simulink model "SIMQGC"  (R2017a)
settings: Solver=VariableStepAuto  StartTime=0.0  StopTime=1000  RelTol=1e-3
model workspace: external: MAT-File (data not in the file)
values from neighbouring files (symbols this model uses):
  aDe =     [MY3.mat]
  aDyn =     [MY3.mat]
  aLat =     [MY3.mat]
  aLon =     [MY3.mat]
  H = HGround + geo.Zgear + GearData.R - MCdata.mass*9.8/4/GearData.Sp    [my3_acdata.m]
  HGround = 500    [my3_acdata.m]
  phi_max = 20    [my3_acdata.m]
  phi_min = -20    [my3_acdata.m]
  psi_max = 30    [my3_acdata.m]
  psi_min = -30    [my3_acdata.m]
  theta_max = 20    [my3_acdata.m]
  theta_min = -20    [my3_acdata.m]
  Xmax = 0.01    [my3_acdata.m]
  Xmin = 0    [my3_acdata.m]
  Ymax = 0.01    [my3_acdata.m]
  Ymin = 0    [my3_acdata.m]
  Zmax = 0.01    [my3_acdata.m]
  Zmin = 0    [my3_acdata.m]
undefined symbols (not defined in the file or in its folder): Earth, geo, ini, magnitude, Motor, Newton, Prop, Raphson, Standard_Devices, UDP_Protocol, WGS84
undefined symbols (not defined in the file): GearData, LProp, RProp
libraries: simulink_extras x12, dspnetwork x8, aerolibobsolete x6, sharedutil x6, simulink x4, aerolibfltsims x3, aerolibasang x2, aerolibatmos2 x1, aerolibbdyn x1, aerolibtransform2 x1, aerolibanimutils x1, sldrtlib x1
(part 1 of 3)
settings Model: Creator=d8230  LastModifiedBy=d8230
settings SFSimCC: SimCustomInitializer=my_3acdata.m
settings RTWCC: Toolchain=Microsoft Visual C++ 2015 v14.0 | nmake (64-bit Windows)
settings CodeAppCC: ForceParamTrailComments=on  MATLABSourceComments=on

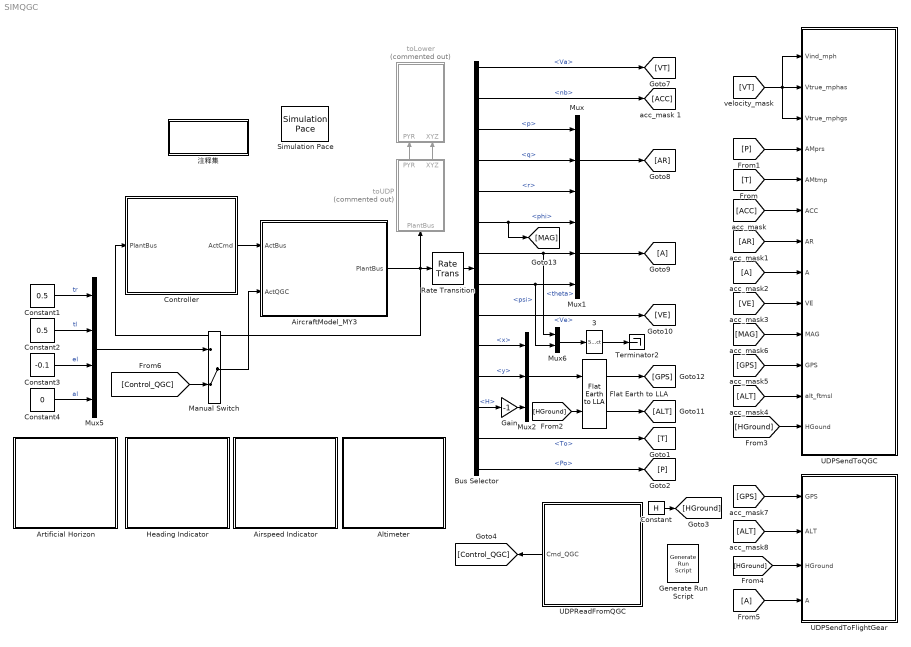
== system SIMQGC ==
  3 : Selector  InputPortWidth=2  IndexOptions=Index vector (dialog)  Indices=[2,1]  OutputSizes=1
  AircraftModel_MY3 : Subsystem
  Airspeed Indicator : Subsystem  DialogController=aeroblksHMICreateDDGDialog  IsWebBlock=on  mask(MWDashboardBlock){webBlockId=530eda5d-0ac3-4735-9d39-42895928f7ce, webBlockType=airspeedindicator, ShowInLibBrowser=on, ShowInitialText=on, HMISrcModelName=SIMQGC}
      mask prompts: webBlockId "WebBlock Id"; webBlockType "WebBlock Type"; HMISrcModelName "Source Model"
      mask help: aeroblksHMI:aeroblkhmi:AirspeedIndicatorDialogDesc
      mask Help: eval('asbhmihelp(''airspeedindicator'')');
      mask Display:
      | if strcmp(get_param(bdroot(gcb),'BlockDiagramType'), 'library')
      |  image([(matlabroot) '/toolbox/aeroblks/aeroblks/hmi/icons/AirspeedIndicatorIcon.svg'])
      | end
  Altimeter : Subsystem  DialogController=aeroblksHMICreateDDGDialog  IsWebBlock=on  mask(MWDashboardBlock){webBlockId=e81fc4a0-2f3e-46f7-8fff-bae700747e07, webBlockType=altimeter, ShowInLibBrowser=on, ShowInitialText=on, HMISrcModelName=SIMQGC}
      mask prompts: webBlockId "WebBlock Id"; webBlockType "WebBlock Type"; HMISrcModelName "Source Model"
      mask help: aeroblksHMI:aeroblkhmi:AltimeterDialogDesc
      mask Help: eval('asbhmihelp(''altimeter'')');
      mask Display:
      | if strcmp(get_param(bdroot(gcb),'BlockDiagramType'), 'library')
      |  image([(matlabroot) '/toolbox/aeroblks/aeroblks/hmi/icons/AltimeterIcon.svg'])
      | end
  Artificial Horizon : Subsystem  DialogController=aeroblksHMICreateDDGDialog  IsWebBlock=on  mask(MWDashboardBlock){webBlockId=e4013b59-c6b3-40ec-8031-c9c080829948, webBlockType=artificialhorizon, ShowInLibBrowser=on, ShowInitialText=on, HMISrcModelName=SIMQGC}
      mask prompts: webBlockId "WebBlock Id"; webBlockType "WebBlock Type"; HMISrcModelName "Source Model"
      mask help: aeroblksHMI:aeroblkhmi:ArtificialHorizonDialogDesc
      mask Help: eval('asbhmihelp(''artificialhorizon'')');
      mask Display:
      | if strcmp(get_param(bdroot(gcb),'BlockDiagramType'), 'library')
      |  image([(matlabroot) '/toolbox/aeroblks/aeroblks/hmi/icons/ArtificialHorizonIcon.svg'])
      | end
  Bus Selector : BusSelector  OutputSignals=Va,nb,p,q,r,phi,theta,psi,Ve,x,y,H,To,Po
  Constant : Constant  Value=H
  Constant1 : Constant  Value=0.5
  Constant2 : Constant  Value=0.5
  Constant3 : Constant  Value=-0.1
  Constant4 : Constant  Value=0
  Controller : Subsystem
  Flat Earth to LLA : aerolibtransform2/Flat Earth to LLA  units=Metric (MKS)  ptype=Earth (WGS84)  F=1/298.257223563  R=6378137  LL0=[34.3,108.80]  psi=0
  Gain : Gain  Gain=-1
  Generate Run Script : aerolibfltsims/Generate Run Script  OutputFileName=runfg.bat  FlightGearBaseDirectory=D:\FlightGear 3.4.0  GeometryModelName=c172p  DestinationPort=6666  OriginAddress=127.0.0.1  OriginPort=5505  LocalAddress=127.0.0.1  AirportId=KSFO  RunwayId=10L  InitialAltitude=ini.Xe(3)/0.3048  InitialHeading=0  OffsetDistance=0  OffsetAzimuth=0  GenerateFile=off  Architecture=Win64  dataFlow=Send
  Heading Indicator : Subsystem  DialogController=aeroblksHMICreateDDGDialog  IsWebBlock=on  mask(MWDashboardBlock){webBlockId=3416712c-36e7-4a0f-be9c-29638a8fd49d, webBlockType=headingindicator, ShowInLibBrowser=on, ShowInitialText=on, HMISrcModelName=SIMQGC}
      mask prompts: webBlockId "WebBlock Id"; webBlockType "WebBlock Type"; HMISrcModelName "Source Model"
      mask help: aeroblksHMI:aeroblkhmi:HeadingIndicatorDialogDesc
      mask Help: eval('asbhmihelp(''headingindicator'')');
      mask Display:
      | if strcmp(get_param(bdroot(gcb),'BlockDiagramType'), 'library')
      |  image([(matlabroot) '/toolbox/aeroblks/aeroblks/hmi/icons/HeadingIndicatorIcon.svg'])
      | end
  Manual Switch : ManualSwitch  CurrentSetting=0
  Mux : Mux  Inputs=3
  Mux1 : Mux  Inputs=3
  Mux2 : Mux  Inputs=3
  Mux5 : Mux
  Mux6 : Mux  Inputs=2
  Rate Transition : RateTransition  OutPortSampleTime=0.05
  Simulation Pace : aerolibanimutils/Simulation Pace  SimulationPace=1  SleepMode=MATLAB Thread  OutputPaceError=off  SampleTime=1/30
  Terminator2 : Terminator
  UDPReadFromQGC : Subsystem
  UDPSendToFlightGear : Subsystem
  UDPSendToQGC : Subsystem
  toLower : Subsystem  Commented=on
  toUDP : Subsystem  Commented=on
  注释集 : Subsystem
  wires:
  [P] -> UDPSendToQGC/4(AMprs)
  [T] -> UDPSendToQGC/5(AMtmp)
  [ACC] -> UDPSendToQGC/6(ACC)
  [AR] -> UDPSendToQGC/7(AR)
  [A] -> UDPSendToQGC/8(A)
  [VE] -> UDPSendToQGC/9(VE)
  [MAG] -> UDPSendToQGC/10(MAG)
  [GPS] -> UDPSendToQGC/11(GPS)
  [ALT] -> UDPSendToQGC/12(alt_ftmsl)
  [VT] -> UDPSendToQGC/1(Vind_mph), UDPSendToQGC/2(Vtrue_mphas), UDPSendToQGC/3(Vtrue_mphgs)
  Mux/1 -> [AR]
  Bus Selector/12 -> Gain/1  "<H>"
  Mux1/1 -> [A]
  Flat Earth to LLA/1 -> [GPS]
  Bus Selector/1 -> [VT]  "<Va>"
  Bus Selector/2 -> [ACC]  "<nb>"
  Bus Selector/3 -> Mux/1  "<p>"
  Bus Selector/4 -> Mux/2  "<q>"
  Bus Selector/5 -> Mux/3  "<r>"
  Bus Selector/6 -> Mux1/1, [MAG]  "<phi>"
  Bus Selector/7 -> Mux1/2, Mux6/1  "<theta>"
  Bus Selector/8 -> Mux1/3, Mux6/2  "<psi>"
  Bus Selector/9 -> [VE]  "<Ve>"
  Bus Selector/10 -> Mux2/1  "<x>"
  Bus Selector/11 -> Mux2/2  "<y>"
  Controller/1(ActCmd) -> AircraftModel_MY3/1(ActBus)
  Mux2/1 -> Flat Earth to LLA/1
  Flat Earth to LLA/2 -> [ALT]
  Gain/1 -> Mux2/3
  [HGround] -> Flat Earth to LLA/2
  toUDP/2(XYZ) -> toLower/2(XYZ)
  toUDP/1(PYR) -> toLower/1(PYR)
  AircraftModel_MY3/1(PlantBus) -> toUDP/1(PlantBus), Controller/1(PlantBus), Rate Transition/1
  Rate Transition/1 -> Bus Selector/1
  Bus Selector/13 -> [T]  "<To>"
  Bus Selector/14 -> [P]  "<Po>"
  Constant1/1 -> Mux5/1  "tr"
  Constant2/1 -> Mux5/2  "tl"
  Constant3/1 -> Mux5/3  "el"
  Constant/1 -> [HGround]
  [HGround] -> UDPSendToQGC/13("HGound ")
  [GPS] -> UDPSendToFlightGear/1(GPS)
  [ALT] -> UDPSendToFlightGear/2(ALT)
  [HGround] -> UDPSendToFlightGear/3(HGround)
  [A] -> UDPSendToFlightGear/4(A)
  3/1 -> Terminator2/1
  Mux6/1 -> 3/1
  Constant4/1 -> Mux5/4  "al"
  Manual Switch/1 -> AircraftModel_MY3/2(ActQGC)
  Mux5/1 -> Manual Switch/1
  [Control_QGC] -> Manual Switch/2
  UDPReadFromQGC/1(Cmd_QGC) -> [Control_QGC]

== system SIMQGC/AircraftModel_MY3 ==
  ActBus : Inport
  ActQGC : Inport  Port=2
  Actuator : Subsystem
  Actuator1 : Subsystem
  Bus Creator : BusCreator  Inputs=23
  Bus Selector : BusSelector  OutputSignals=dt,de,dd,da
  Constant{,1..3} (4 alike) : Constant  Value=0
  Demux : Demux
  Demux1 : Demux
  Environment : Subsystem  TreatAsAtomicUnit=on
  Fixwing_Airframe : Subsystem  TreatAsAtomicUnit=on
      mask Display:
      | port_label('output',1,'PlantData');
      | port_label('input',1,'EnvmData');
      | port_label('input',2,'ActData');
  Manual Switch : ManualSwitch  CurrentSetting=0
  Scope1 : Scope  NumInputPorts=4
  Scopes : Subsystem
  Terminator{,1..3} (4 alike) : Terminator
  outputs : Subsystem
  PlantBus : Outport
  wires:
  ActBus/1 -> Bus Selector/1
  Bus Selector/2 -> Actuator/2(de_cmd)  "<de>"
  Fixwing_Airframe/1(PlantData) -> outputs/1(Model o/p bus), Scopes/1(plant bus)
  outputs/1(p) -> Terminator3/1  "p"
  Bus Selector/3 -> Actuator/3(dd_cmd)  "<dd>"
  Environment/1(Envm) -> Fixwing_Airframe/1(EnvmData)
  Actuator/1(Airc) -> Manual Switch/1
  Bus Selector/1 -> Actuator/1(dt_cmd)  "<dt>"
  Bus Creator/1 -> PlantBus/1
  outputs/2(q) -> Bus Creator/2  "q"
  outputs/3(r) -> Terminator1/1  "r"
  outputs/4(phi) -> Terminator2/1  "phi"
  outputs/5(theta) -> Bus Creator/5  "theta"
  outputs/6(psi) -> Terminator/1  "psi"
  outputs/7(alpha) -> Bus Creator/7  "alpha"
  outputs/8(beta) -> Bus Creator/8  "beta"
  outputs/9(Va) -> Bus Creator/9  "Va"
  outputs/10(x) -> Bus Creator/10  "x"
  outputs/11(y) -> Bus Creator/11  "y"
  outputs/12(H) -> Bus Creator/12, Environment/1(H)  "H"
  outputs/13(mach) -> Bus Creator/13  "mach"
  outputs/14(gamma) -> Bus Creator/14  "gamma"
  outputs/15(chi) -> Bus Creator/15  "chi"
  outputs/16(Vy) -> Bus Creator/16  "Vy"
  outputs/17(nyb) -> Bus Creator/17  "nyb"
  outputs/18(nzb) -> Bus Creator/18  "nzb"
  outputs/19(Acc) -> Bus Creator/19  "Acc"
  outputs/20(Ve) -> Bus Creator/20  "Ve"
  ActQGC/1 -> Demux/1
  outputs/21(To) -> Bus Creator/21
  outputs/22(Po) -> Bus Creator/22
  Demux/1 -> Actuator1/1(tr_cmd)
  Demux/2 -> Actuator1/2(tl_cmd)
  Actuator1/1(Airc) -> Manual Switch/2
  Manual Switch/1 -> Demux1/1, Fixwing_Airframe/2(ActData)
  Bus Selector/4 -> Actuator/4(da_cmd)  "<da>"
  Demux/4 -> Actuator1/4(al_cmd)
  Constant/1 -> Bus Creator/6  "psi"
  Constant1/1 -> Bus Creator/3  "r"
  Constant2/1 -> Bus Creator/1  "p"
  Constant3/1 -> Bus Creator/4  "phi"
  Demux1/1 -> Scope1/1
  Demux1/2 -> Scope1/2
  Demux1/3 -> Scope1/3
  Demux1/4 -> Scope1/4
  Demux/3 -> Actuator1/3(el_cmd)
  outputs/23(nb) -> Bus Creator/23

== system SIMQGC/Airspeed Indicator ==

== system SIMQGC/Altimeter ==

== system SIMQGC/Artificial Horizon ==

== system SIMQGC/Controller ==
  PlantBus : Inport
  Add : Sum  Inputs=|+-
  Bus Creator : BusCreator  Inputs=4
  Bus Selector : BusSelector  OutputSignals=Va,gamma,H,theta,q,y,phi,p,nyb,r,psi
  Constant : Constant  Value=0
  Constant1 : Constant  Value=0
  Constant2 : Constant  Value=-600
  Gain{1,3..5} (4 alike) : Gain  Gain=1/57.3
  Gain2 : Gain  Gain=9.8
  Gain6 : Gain
  MATLAB Function : MATLAB Function  TreatAsAtomicUnit=on
  Memory1 : Memory
  RAH : Subsystem  mask{Kphi=1, Kp=3, Kr=1.4, Kff_phi=0.2, Kay=0, Kpi=0.5}
  Subsystem : Subsystem
  Terminator : Terminator
  Terminator1 : Terminator
  height_hold : Subsystem
  theta_hold : Subsystem
  v_hold1 : Subsystem
  ActCmd : Outport
  wires:
  Bus Creator/1 -> ActCmd/1  "ActCmd"
  PlantBus/1 -> Bus Selector/1
  v_hold1/1(tg) -> [dt]  "dt"
  theta_hold/1(de) -> [de]  "de"
  Bus Selector/1 -> v_hold1/1(Va)  "<Va>"
  Bus Selector/4 -> theta_hold/2(theta)  "<theta>"
  Bus Selector/5 -> theta_hold/3(q)  "<q>"
  Constant/1 -> v_hold1/2(Vc)
  height_hold/1(thetac) -> theta_hold/1(thetac)
  Bus Selector/3 -> MATLAB Function/1(H), height_hold/1(Hc)  "<H>"
  Bus Selector/7 -> Gain3/1  "<phi>"
  Bus Selector/8 -> Gain1/1  "<p>"
  Bus Selector/10 -> Gain4/1  "<r>"
  Bus Selector/9 -> Gain2/1  "<nyb>"
  RAH/1(dd) -> Memory1/1  "dd"
  Bus Selector/2 -> Terminator/1  "<gamma>"
  Bus Selector/6 -> Terminator1/1  "<y>"
  Gain2/1 -> RAH/5(ayb)
  Gain1/1 -> RAH/3(p)
  Gain3/1 -> RAH/2(phi)
  Gain4/1 -> RAH/4(r)
  Gain5/1 -> RAH/1(Phic)
  Gain6/1 -> [dd]  "dd"
  Constant2/1 -> height_hold/2(H)
  MATLAB Function/1(phic) -> Gain5/1
  [dt] -> Bus Creator/1  "dt"
  [de] -> Bus Creator/2  "de"
  [dd] -> Bus Creator/3  "dd"
  [da] -> Bus Creator/4  "da"
  Constant1/1 -> Add/2
  Bus Selector/11 -> Add/1  "<psi>"
  Memory1/1 -> Gain6/1
  Add/1 -> Subsystem/1(In1)
  Subsystem/1(Out1) -> [da]

== system SIMQGC/Heading Indicator ==

== system SIMQGC/UDPReadFromQGC ==
  Mux4 : Mux
  Subsystem : Subsystem
  Terminator4 : Terminator
  UDP Receive : dspnetwork/UDP Receive  localURL='0.0.0.0'  localPort=59000  remoteURL='127.0.0.1'  remotePort=-1  recvBufferSize=8192  dims=41  signalDatatype=uint8  isVarSize=off  showBlockingTime=off  blockingTime=0  sampletime=0.02  blockPlatform=[]
  Cmd_QGC : Outport
  wires:
  Subsystem/3(elev_yoke) -> Mux4/3
  Subsystem/1(thro1_part) -> Mux4/1
  Subsystem/5(ruddr_yoke) -> Terminator4/1
  UDP Receive/1 -> Subsystem/1(msg)
  Subsystem/2(thro2_part) -> Mux4/2
  Mux4/1 -> Cmd_QGC/1
  Subsystem/4(ailrn_yoke) -> Mux4/4
  UDP Receive/2 -> Subsystem/2(length)

== system SIMQGC/UDPSendToFlightGear ==
  GPS : Inport
  ALT : Inport  Port=2
  HGround : Inport  Port=3
  A : Inport  Port=4
  3 : Selector  InputPortWidth=2  IndexOptions=Index vector (dialog)  Indices=[2,1]  OutputSizes=1
  Add : Sum
  Constant : Constant  Value=0
  Data Type Conversion2 : DataTypeConversion  OutDataTypeStr=single
  Demux : Demux  Outputs=3
  Demux1 : Demux  Outputs=2
  Gain1 : Gain  Gain=pi/180
  Manual Switch : ManualSwitch  CurrentSetting=0
  Pack net_fdm Packet for FlightGear : aerolibfltsims/Pack net_fdm Packet for FlightGear  FlightGearVersion=v3.4  ShowPositionAttitudeInputs=on  ShowVelocityAccelerationInputs=off  ShowControlSurfacePositionInputs=off  ShowEngineFuelInputs=off  ShowLandingGearInputs=off  ShowEnvironmentInputs=off  SampleTime=-1
      settings: SourceProductName=Aerospace Blockset  SourceProductBaseCode=AE
  Send net_fdm Packet to FlightGear : aerolibfltsims/Send net_fdm Packet to FlightGear  DestinationIpAddress=127.0.0.1  DestinationPort=6666  LocalIpPort=-1  varLen=off  SampleTime=-1
      settings: SourceProductName=Aerospace Blockset  SourceProductBaseCode=AE
  Unit Conversion : UnitConversion
  wires:
  A/1 -> Gain1/1
  Pack net_fdm Packet for FlightGear/1 -> Send net_fdm Packet to FlightGear/1
  Demux/2 -> Pack net_fdm Packet for FlightGear/5
  Demux/3 -> Pack net_fdm Packet for FlightGear/6
  ALT/1 -> Add/1
  HGround/1 -> Manual Switch/1
  Demux/1 -> Pack net_fdm Packet for FlightGear/4
  Add/1 -> Pack net_fdm Packet for FlightGear/3
  GPS/1 -> Unit Conversion/1
  3/1 -> Demux1/1
  Data Type Conversion2/1 -> Demux/1
  Constant/1 -> Manual Switch/2
  Manual Switch/1 -> Add/2
  Gain1/1 -> Data Type Conversion2/1
  Demux1/1 -> Pack net_fdm Packet for FlightGear/1
  Demux1/2 -> Pack net_fdm Packet for FlightGear/2
  Unit Conversion/1 -> 3/1

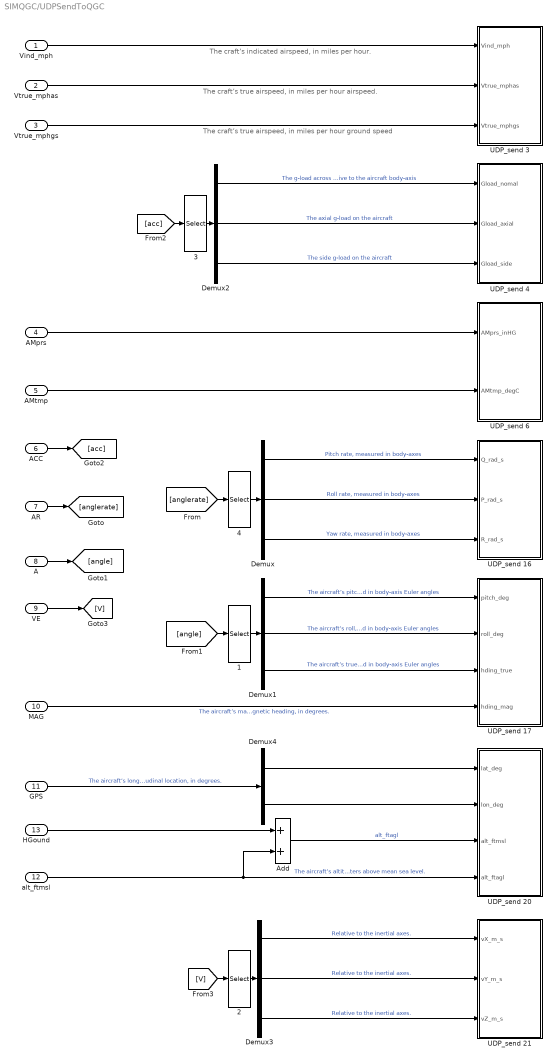
== system SIMQGC/UDPSendToQGC ==
  note: The craft’s indicated airspeed, in miles per hour.
  note: The craft’s true airspeed, in miles per hour airspeed.
  note: The craft’s true airspeed, in miles per hour ground speed
  Vind_mph : Inport
  Vtrue_mphas : Inport  Port=2
  Vtrue_mphgs : Inport  Port=3
  AMprs : Inport  Port=4
  AMtmp : Inport  Port=5
  ACC : Inport  Port=6
  AR : Inport  Port=7
  A : Inport  Port=8
  VE : Inport  Port=9
  MAG : Inport  Port=10
  GPS : Inport  Port=11
  alt_ftmsl : Inport  Port=12
  "HGound " : Inport  Port=13
  1 : Selector  InputPortWidth=3  IndexOptions=Index vector (dialog)  Indices=[2,3,1]  OutputSizes=1
  2 : Selector  InputPortWidth=3  IndexOptions=Index vector (dialog)  Indices=[2,3,1]  OutputSizes=1
  3 : Selector  InputPortWidth=3  IndexOptions=Index vector (dialog)  Indices=[3,1,2]  OutputSizes=1
  4 : Selector  InputPortWidth=3  IndexOptions=Index vector (dialog)  Indices=[2,1,3]  OutputSizes=1
  Add : Sum
  Demux{,1..3} (4 alike) : Demux  Outputs=3
  Demux4 : Demux  Outputs=2
  UDP_send 16 : Subsystem
  UDP_send 17 : Subsystem
  UDP_send 20 : Subsystem
  UDP_send 21 : Subsystem
  "UDP_send 3 " : Subsystem
  UDP_send 4 : Subsystem
  UDP_send 6 : Subsystem
  wires:
  AMtmp/1 -> UDP_send 6/2(AMtmp_degC)
  Demux2/1 -> UDP_send 4/1(Gload_nomal)  "The g-load across the aircraft, relative to the aircraft body-axis"
  Demux2/2 -> UDP_send 4/2(Gload_axial)  "The axial g-load on the aircraft"
  Vtrue_mphgs/1 -> "UDP_send 3 "/3(Vtrue_mphgs)
  Vind_mph/1 -> "UDP_send 3 "/1(Vind_mph)
  Vtrue_mphas/1 -> "UDP_send 3 "/2(Vtrue_mphas)
  AR/1 -> [anglerate]
  [angle] -> 1/1
  ACC/1 -> [acc]
  [acc] -> 3/1
  AMprs/1 -> UDP_send 6/1(AMprs_inHG)
  Demux/3 -> UDP_send 16/3(R_rad_s)  "Yaw rate, measured in body-axes"
  Demux/2 -> UDP_send 16/2(P_rad_s)  "Roll rate, measured in body-axes"
  MAG/1 -> UDP_send 17/4(hding_mag)  "The aircraft’s magnetic heading, in degrees."
  GPS/1 -> Demux4/1  "The aircraft’s longitudinal location, in degrees."
  alt_ftmsl/1 -> Add/2, UDP_send 20/4(alt_ftagl)  "The aircraft’s altitude, in meters above mean sea level."
  [anglerate] -> 4/1
  Demux1/2 -> UDP_send 17/2(roll_deg)  "The aircraft’s roll, measured in body-axis Euler angles"
  Demux1/3 -> UDP_send 17/3(hding_true)  "The aircraft’s true heading, measured in body-axis Euler angles"
  Demux1/1 -> UDP_send 17/1(pitch_deg)  "The aircraft’s pitch, measured in body-axis Euler angles"
  Demux3/1 -> UDP_send 21/1(vX_m_s)  "Relative to the inertial axes."
  Demux3/2 -> UDP_send 21/2(vY_m_s)  "Relative to the inertial axes."
  Demux3/3 -> UDP_send 21/3(vZ_m_s)  "Relative to the inertial axes."
  Demux/1 -> UDP_send 16/1(Q_rad_s)  "Pitch rate, measured in body-axes"
  [V] -> 2/1
  VE/1 -> [V]
  A/1 -> [angle]
  Demux2/3 -> UDP_send 4/3(Gload_side)  "The side g-load on the aircraft"
  Demux4/1 -> UDP_send 20/1(lat_deg)
  Demux4/2 -> UDP_send 20/2(lon_deg)
  4/1 -> Demux/1
  1/1 -> Demux1/1
  "HGound "/1 -> Add/1
  Add/1 -> UDP_send 20/3(alt_ftmsl)  "alt_ftagl"
  2/1 -> Demux3/1
  3/1 -> Demux2/1

== system SIMQGC/toLower ==
  PYR : Inport
  XYZ : Inport  Port=2
  Constant : Constant  Value=777  OutDataTypeStr=int32
  Constant1 : Constant  Value=5  OutDataTypeStr=int32
  Constant7 : Constant  Value=10
  Constant8 : Constant  Value=0
  Demux : Demux  Outputs=3
  Demux1 : Demux  Outputs=3
  Packet Output : sldrtlib/Packet Output  SampleTime=0.01  MaxMissedTicks=50  ShowMissedTicks=off  YieldWhenWaiting=off  DrvName=Standard_Devices/UDP_Protocol  DrvAddress=9000  DrvOptions=[3232235877 9001]  PacketSize=72  DataTypes={'int32','int32','double','double','double','double','double','double','double','double'}  ShowReady=off  ShowError=off  PacketID=1  ByteOrder=1  InitialValue=[]  FinalValue=[]
      settings: AttributesFormatString=Standard Devices\nUDP Protocol [2328h]  SourceProductName=Simulink Desktop Real-Time
  Rate Transition : RateTransition  OutPortSampleTime=0.01
  Rate Transition1 : RateTransition  OutPortSampleTime=0.01
  wires:
  Constant8/1 -> Packet Output/10
  Constant/1 -> Packet Output/1
  Constant7/1 -> Packet Output/9
  Demux/1 -> Packet Output/3
  Demux/2 -> Packet Output/4
  Demux/3 -> Packet Output/5
  Constant1/1 -> Packet Output/2
  Demux1/1 -> Packet Output/6
  Demux1/2 -> Packet Output/7
  Demux1/3 -> Packet Output/8
  XYZ/1 -> Rate Transition1/1
  PYR/1 -> Rate Transition/1
  Rate Transition/1 -> Demux/1
  Rate Transition1/1 -> Demux1/1

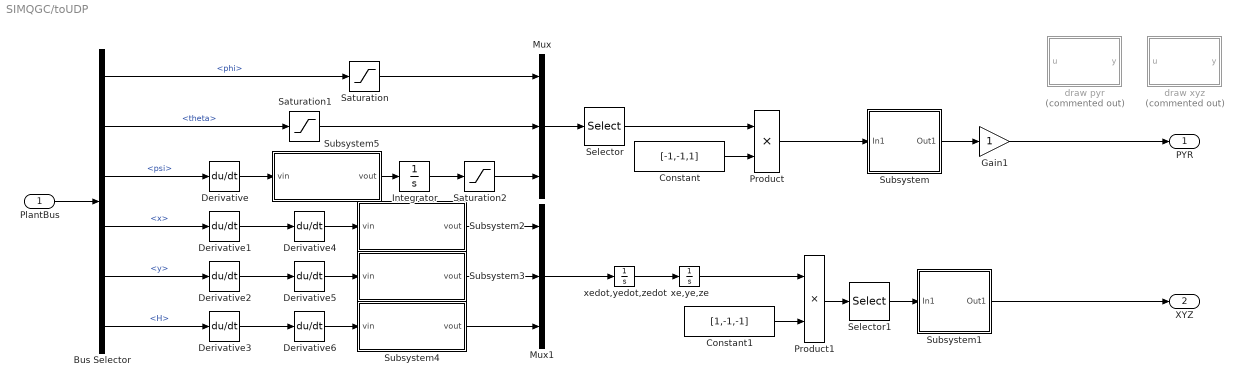
== system SIMQGC/toUDP ==
  PlantBus : Inport
  Bus Selector : BusSelector  OutputSignals=phi,theta,psi,x,y,H
  Constant : Constant  Value=[-1,-1,1]
  Constant1 : Constant  Value=[1,-1,-1]
  Derivative{,1..6} (7 alike) : Derivative
  Gain1 : Gain
  Integrator : Integrator
  Mux : Mux  Inputs=3
  Mux1 : Mux  Inputs=3
  Product : Product
  Product1 : Product
  Saturation : Saturate  UpperLimit=phi_max  LowerLimit=phi_min
  Saturation1 : Saturate  UpperLimit=theta_max  LowerLimit=theta_min
  Saturation2 : Saturate  UpperLimit=psi_max  LowerLimit=psi_min
  Selector : Selector  InputPortWidth=3  IndexOptions=Index vector (dialog)  Indices=[2,3,1]  OutputSizes=1
  Selector1 : Selector  InputPortWidth=3  IndexOptions=Index vector (dialog)  Indices=[2,3,1]  OutputSizes=1
  Subsystem : Subsystem
  Subsystem1 : Subsystem
  Subsystem2 : Subsystem  mask{t=1}
      mask prompts: t "Threshhold"
  Subsystem3 : Subsystem  mask{t=1}
      mask prompts: t "Threshhold"
  Subsystem4 : Subsystem  mask{t=1}
      mask prompts: t "Threshhold"
  Subsystem5 : Subsystem  mask{t=1}
      mask prompts: t "Threshhold"
  draw pyr : MATLAB Function  Commented=on  TreatAsAtomicUnit=on
  draw xyz : MATLAB Function  Commented=on  TreatAsAtomicUnit=on
  xe,ye,ze : Integrator  InitialCondition=[0,0,0]  LimitOutput=on  UpperSaturationLimit=[Xmax,Ymax,Zmax]  LowerSaturationLimit=[Xmin,Ymin,Zmin]
  xedot,yedot,zedot : Integrator  InitialCondition=[0,0,0]  UpperSaturationLimit=[Xmax,Ymax,Zmax]  LowerSaturationLimit=[Xmin,Ymin,Zmin]
  PYR : Outport
  XYZ : Outport  Port=2
  wires:
  PlantBus/1 -> Bus Selector/1
  Selector/1 -> Product/1
  xe,ye,ze/1 -> Product1/1
  Product1/1 -> Selector1/1
  Constant1/1 -> Product1/2
  Constant/1 -> Product/2
  Product/1 -> Subsystem/1(In1)
  Subsystem/1(Out1) -> Gain1/1
  Selector1/1 -> Subsystem1/1(In1)
  Bus Selector/3 -> Derivative/1  "<psi>"
  Derivative/1 -> Subsystem5/1(vin)
  Bus Selector/1 -> Saturation/1  "<phi>"
  Bus Selector/2 -> Saturation1/1  "<theta>"
  Subsystem5/1(vout) -> Integrator/1
  Mux/1 -> Selector/1
  Integrator/1 -> Saturation2/1
  Bus Selector/4 -> Derivative1/1  "<x>"
  Bus Selector/5 -> Derivative2/1  "<y>"
  Bus Selector/6 -> Derivative3/1  "<H>"
  Derivative1/1 -> Derivative4/1
  Derivative2/1 -> Derivative5/1
  Derivative3/1 -> Derivative6/1
  Derivative4/1 -> Subsystem2/1(vin)
  Derivative5/1 -> Subsystem3/1(vin)
  Derivative6/1 -> Subsystem4/1(vin)
  Subsystem2/1(vout) -> Mux1/1
  Subsystem3/1(vout) -> Mux1/2
  Subsystem4/1(vout) -> Mux1/3
  Mux1/1 -> xedot,yedot,zedot/1
  xedot,yedot,zedot/1 -> xe,ye,ze/1
  Saturation/1 -> Mux/1
  Saturation1/1 -> Mux/2
  Saturation2/1 -> Mux/3
  Gain1/1 -> PYR/1
  Subsystem1/1(Out1) -> XYZ/1

== system SIMQGC/注释集 ==
  note: 类层次结构
      | LinkManager，LinkInterface
      | QGC中的“链接”是与vehicle 的特定类型的通信管道，例如串口或WiFi上的UDP。所有链接的基类是LinkInterface。每个链接运行在它自己的线程上并发送字节到MAVLinkProtocol。
      | 该LinkManager对象跟踪系统中所有打开的链接。LinkManager还通过串口和UDP链接管理自动连接。
      | MAVLinkProtocol
      | 系统中只有一个MAVLinkProtocol对象。它的任务是从一个链接获取传入的字节并将它们转换为MAVLink消息。MAVLink HEARTBEAT消息被发送到MultiVehicleManager。所有MAVLink消息都被发送到与链路关联的vehicle。
      | MultiVehicleManager
      | 系统中有一个MultiVehicleManager对象。当它在以前没有看到的链接上收到HEARTBEAT时，它会创建一个Vehicle对象。`MultiVehicleManager还可以跟踪系统中的所有vehicle，并处理从一辆活动的vehicle到另一个的切换，并正确处理正在移除的vehicle。
      | Vehicle
      | Vehicle对象是QGC代码通过其与物理设备通信的主接口。
      | 注意：还有一个与每个Vehicle相关的UAS对象，这是一个弃用的类，正在慢慢地逐步淘汰，所有的功能都转移到Vehicle类。这里不应该添加新的代码。
      | FirmwarePlugin，FirmwarePluginManager
      | FirmwarePlugin类被用作固件插件的基类。固件插件包含特定于固件的代码，这样Vehicle对象就是干净的，支持UI的单个标准接口。
      | FirmwarePluginManager是一个工厂类，它根据vehicle的MAV_AUTOPILOT / MAV_TYPE组合创建一个FirmwarePlugin实例。
      | 用户界面设计
      | QGC中UI设计的主要模式是用QML编写的UI页面，多次与用C ++编写的定制“控制器”进行通信。类似MVC的设计模式。
      | QML代码通过以下机制绑定到与系统相关的信息：
      | 自定义控制器
      | QGroundControl提供访问活动Vehicle对象的全局对象
      | FactSystem提供对参数的访问，并且在某些情况下提供自定义Facts
      | 注意：由于QGC中使用的QML的复杂性以及它依赖与C ++对象的通信来驱动ui，所以不可能使用Qt提供的QML Designer来编辑QML。

== system SIMQGC/AircraftModel_MY3/Actuator ==
  dt_cmd : Inport
  de_cmd : Inport  Port=2
  dd_cmd : Inport  Port=3
  da_cmd : Inport  Port=4
  Bus Creator : BusCreator  Inputs=4
  Degrees to Radians : simulink_extras/Transformations/Degrees to Radians
  Sum : Sum  Inputs=|++
  Sum1 : Sum  Inputs=+-|
  Sum2 : Sum  Inputs=|++
  Terminator : Terminator
  Airc : Outport
  wires:
  Bus Creator/1 -> Airc/1
  de_cmd/1 -> Degrees to Radians/1
  dt_cmd/1 -> Sum1/1, Sum2/1, Sum/1  "dt"
  dd_cmd/1 -> Sum1/2, Sum2/2, Sum/2
  Degrees to Radians/1 -> Bus Creator/3  "de"
  Sum1/1 -> Terminator/1  "dtl"
  Sum/1 -> Bus Creator/1  "dtr"
  da_cmd/1 -> Bus Creator/4  "da"
  Sum2/1 -> Bus Creator/2  "dtl"

== system SIMQGC/AircraftModel_MY3/Actuator1 ==
  tr_cmd : Inport
  tl_cmd : Inport  Port=2
  el_cmd : Inport  Port=3
  al_cmd : Inport  Port=4
  Bus Creator : BusCreator  Inputs=4
  Gain : Gain  Gain=-15
  Gain1 : Gain  Gain=10
  Gain2 : Gain  Gain=10
  Airc : Outport
  wires:
  Bus Creator/1 -> Airc/1
  el_cmd/1 -> Gain/1
  tr_cmd/1 -> Gain1/1
  tl_cmd/1 -> Gain2/1
  Gain/1 -> Bus Creator/3  "de"
  al_cmd/1 -> Bus Creator/4  "da"
  Gain1/1 -> Bus Creator/1  "dtr"
  Gain2/1 -> Bus Creator/2  "dtl"

== system SIMQGC/AircraftModel_MY3/Environment ==
  H : Inport
  COESA Atmosphere Model : aerolibatmos2/COESA Atmosphere Model  units=Metric (MKS)  spec=1976 COESA-extended U.S. Standard Atmosphere  model=Profile  profile_var=High temperature  profile_percent=1%  profile_alt=5 km (16404 ft)  envelope_var=High temperature  envelope_percent=1%  action=Warning
  EnvBus : BusCreator  Inputs=8
  Latitude : Constant  Value=34.3
  Memory : Memory  X0=-ini.Xe(3)
  Saturation : Saturate  UpperLimit=80000  LowerLimit=0
  WGS84 Gravity Model : aerolibobsolete/WGS84 Gravity Model  model=WGS84 Taylor Series  units=Metric (MKS)  no_atmos=on  precessing=on  month=February  day=1  year=2000  no_centrifugal=on  action=Warning
      settings: SourceProductName=Aerospace Blockset  SourceProductBaseCode=AE
  c : Constant  Value=0
  c1 : Constant  Value=[0 0 0]
  c2 : Constant  Value=[0 0 0]
  Envm : Outport
  wires:
  EnvBus/1 -> Envm/1  "EnvBus"
  Latitude/1 -> WGS84 Gravity Model/2
  H/1 -> Memory/1
  Saturation/1 -> COESA Atmosphere Model/1, WGS84 Gravity Model/1
  c/1 -> EnvBus/1  "hground"
  c1/1 -> EnvBus/2  "WindVelocity"
  c2/1 -> EnvBus/3  "WindAngleRates"
  COESA Atmosphere Model/1 -> EnvBus/4  "To"
  COESA Atmosphere Model/2 -> EnvBus/5  "a"
  COESA Atmosphere Model/3 -> EnvBus/6  "Po"
  COESA Atmosphere Model/4 -> EnvBus/7  "AirDensity"
  WGS84 Gravity Model/1 -> EnvBus/8  "g"
  Memory/1 -> Saturation/1

== system SIMQGC/AircraftModel_MY3/Fixwing_Airframe ==
  EnvmData : Inport
  ActData : Inport  Port=2
  6DoF (Euler Angles) : aerolibobsolete/6DoF (Euler Angles)  units=Metric (MKS)  mtype=Fixed  rep=Euler Angles  xme_0=ini.Xe  Vm_0=ini.Vb  eul_0=ini.euler  pm_0=ini.pqr  mass_0=ini.mass  mass_e=0.5  mass_f=2.0  inertia=ini.inertia  inertia_e=eye(3)  inertia_f=2*eye(3)  k_quat=1.0
      settings: SourceProductName=Aerospace Blockset  SourceProductBaseCode=AE
  Aerodynamics : Subsystem
  Demux1 : Demux  Outputs=[3,3]
  Gravity : Subsystem
  GroundForces : Subsystem
  PlantBus : Subsystem
  Propulsion : Subsystem
  Sum1 : Sum  Inputs=++++  SaturateOnIntegerOverflow=on
  PlantData : Outport
  wires:
  PlantBus/1(Data) -> GroundForces/1(PlantData), Gravity/1(PlantData), Propulsion/2(PlantData), Aerodynamics/1(PlantData), PlantData/1
  ActData/1 -> Propulsion/1(ActData), Aerodynamics/3(ActData), [ACTData]
  EnvmData/1 -> Propulsion/3(EnvData), [EnvmData], Aerodynamics/2(EnvmData)
  Sum1/1 -> Demux1/1
  6DoF (Euler Angles)/1 -> PlantBus/1(Ve)  "Ve"
  6DoF (Euler Angles)/2 -> PlantBus/2(Xe)  "Xe"
  6DoF (Euler Angles)/3 -> PlantBus/3(Euler)  "Euler"
  6DoF (Euler Angles)/4 -> PlantBus/4(DCM)  "DCM"
  6DoF (Euler Angles)/5 -> PlantBus/5(Vb)  "Vb"
  6DoF (Euler Angles)/6 -> PlantBus/6(pqr)  "pqr"
  6DoF (Euler Angles)/7 -> PlantBus/7(pqrdot)  "pqrdot"
  6DoF (Euler Angles)/8 -> PlantBus/8(Accels)  "Accels"
  [AeroBus] -> PlantBus/9(AeroBus)  "AeroBus"
  [EnvmData] -> PlantBus/10(EnvmData)  "EnvBus"
  [mass] -> PlantBus/11(mass)
  [CG] -> PlantBus/12(CG)
  Gravity/1(FM) -> Sum1/3
  Aerodynamics/2(AeroBus) -> [AeroBus]
  Propulsion/1(FM) -> Sum1/2
  Gravity/2(mass) -> [mass]
  Gravity/3(CG) -> [CG]
  [ACTData] -> PlantBus/13(ACTData)
  GroundForces/2(WOW) -> [WOW]
  [WOW] -> PlantBus/14(WOW)
  Aerodynamics/1(FM) -> Sum1/1
  Demux1/2 -> 6DoF (Euler Angles)/2
  Demux1/1 -> 6DoF (Euler Angles)/1
  GroundForces/1(FM) -> Sum1/4

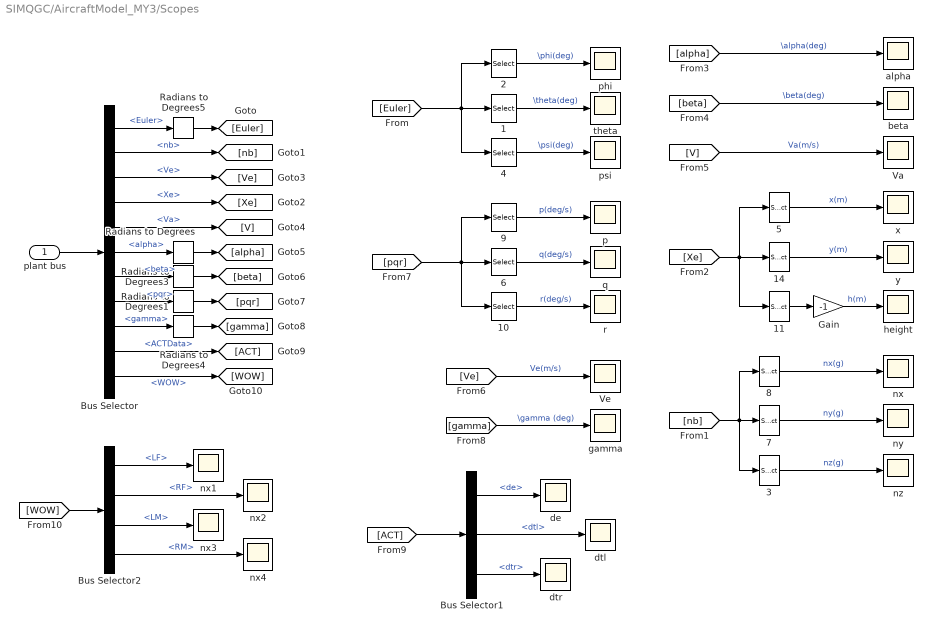
== system SIMQGC/AircraftModel_MY3/Scopes ==
  plant bus : Inport
  {1,6..7,14} (4 alike) : Selector  InputPortWidth=3  IndexOptions=Index vector (dialog)  Indices=2  OutputSizes=1
  {3..4,10..11} (4 alike) : Selector  InputPortWidth=3  IndexOptions=Index vector (dialog)  Indices=3  OutputSizes=1
  {2,5,8..9} (4 alike) : Selector  InputPortWidth=3  IndexOptions=Index vector (dialog)  Indices=1  OutputSizes=1
  Bus Selector : BusSelector  OutputSignals=Euler,nb,Ve,Xe,Va,alpha,beta,pqr,gamma,ACTData,WOW
  Bus Selector1 : BusSelector  OutputSignals=de,dtl,dtr
  Bus Selector2 : BusSelector  OutputSignals=LF,RF,LM,RM
  Gain : Gain  Gain=-1
  Radians to Degrees{,1,3..5} (5 alike) : simulink_extras/Transformations/Radians to Degrees
  Va : Scope
  Ve : Scope
  alpha : Scope
  beta : Scope
  de : Scope
  dtl : Scope
  dtr : Scope
  gamma : Scope
  height : Scope
  nx{,1..4} (5 alike) : Scope
  ny : Scope
  nz : Scope
  p : Scope
  phi : Scope
  psi : Scope
  q : Scope
  r : Scope
  theta : Scope
  x : Scope
  y : Scope
  wires:
  Bus Selector/2 -> [nb]  "<nb>"
  [nb] -> 7/1, 8/1, 3/1
  3/1 -> nz/1  "nz(g)"
  8/1 -> nx/1  "nx(g)"
  7/1 -> ny/1  "ny(g)"
  Radians to Degrees5/1 -> [Euler]
  plant bus/1 -> Bus Selector/1
  1/1 -> theta/1  "\\theta(deg)"
  Bus Selector/4 -> [Xe]  "<Xe>"
  2/1 -> phi/1  "\\phi(deg)"
  4/1 -> psi/1  "\\psi(deg)"
  Bus Selector/6 -> Radians to Degrees/1  "<alpha>"
  [Euler] -> 1/1, 2/1, 4/1
  Bus Selector/1 -> Radians to Degrees5/1  "<Euler>"
  [Xe] -> 5/1, 14/1, 11/1
  Bus Selector/3 -> [Ve]  "<Ve>"
  Bus Selector/5 -> [V]  "<Va>"
  Radians to Degrees/1 -> [alpha]
  Bus Selector/7 -> Radians to Degrees3/1  "<beta>"
  Radians to Degrees3/1 -> [beta]
  [beta] -> beta/1  "\\beta(deg)"
  [alpha] -> alpha/1  "\\alpha(deg)"
  [Ve] -> Ve/1  "Ve(m/s)"
  Bus Selector/8 -> Radians to Degrees1/1  "<pqr>"
  6/1 -> q/1  "q(deg/s)"
  9/1 -> p/1  "p(deg/s)"
  10/1 -> r/1  "r(deg/s)"
  [pqr] -> 10/1, 9/1, 6/1
  Radians to Degrees1/1 -> [pqr]
  11/1 -> Gain/1
  Gain/1 -> height/1  "h(m)"
  5/1 -> x/1  "x(m)"
  Bus Selector/9 -> Radians to Degrees4/1  "<gamma>"
  Radians to Degrees4/1 -> [gamma]
  [gamma] -> gamma/1  "\\gamma (deg)"
  14/1 -> y/1  "y(m)"
  [V] -> Va/1  "Va(m/s)"
  Bus Selector/10 -> [ACT]  "<ACTData>"
  [ACT] -> Bus Selector1/1
  Bus Selector1/1 -> de/1  "<de>"
  Bus Selector1/3 -> dtr/1  "<dtr>"
  Bus Selector/11 -> [WOW]  "<WOW>"
  Bus Selector1/2 -> dtl/1  "<dtl>"
  [WOW] -> Bus Selector2/1
  Bus Selector2/1 -> nx1/1  "<LF>"
  Bus Selector2/2 -> nx2/1  "<RF>"
  Bus Selector2/3 -> nx3/1  "<LM>"
  Bus Selector2/4 -> nx4/1  "<RM>"

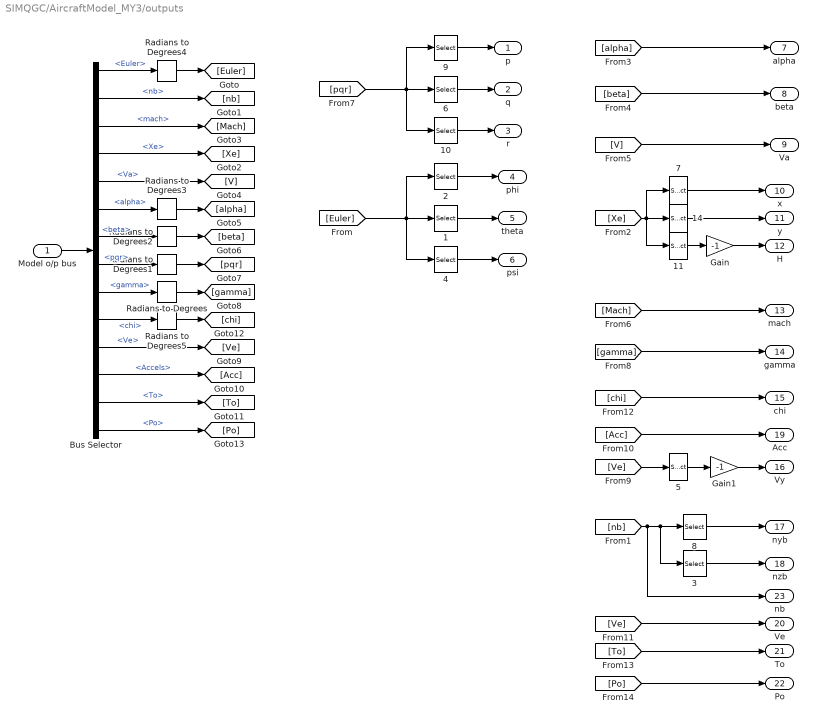
== system SIMQGC/AircraftModel_MY3/outputs ==
  Model o/p bus : Inport
  {1,5..6,8,14} (5 alike) : Selector  InputPortWidth=3  IndexOptions=Index vector (dialog)  Indices=2  OutputSizes=1
  {3..4,10..11} (4 alike) : Selector  InputPortWidth=3  IndexOptions=Index vector (dialog)  Indices=3  OutputSizes=1
  2 : Selector  InputPortWidth=3  IndexOptions=Index vector (dialog)  Indices=1  OutputSizes=1
  7 : Selector  InputPortWidth=3  IndexOptions=Index vector (dialog)  Indices=1  OutputSizes=1
  9 : Selector  InputPortWidth=3  IndexOptions=Index vector (dialog)  Indices=1  OutputSizes=1
  Bus Selector : BusSelector  OutputSignals=Euler,nb,mach,Xe,Va,alpha,beta,pqr,gamma,chi,Ve,Accels,To,Po
  Gain : Gain  Gain=-1
  Gain1 : Gain  Gain=-1
  Radians to Degrees{,1..5} (6 alike) : simulink_extras/Transformations/Radians to Degrees
  p : Outport
  q : Outport  Port=2
  r : Outport  Port=3
  phi : Outport  Port=4
  theta : Outport  Port=5
  psi : Outport  Port=6
  alpha : Outport  Port=7
  beta : Outport  Port=8
  Va : Outport  Port=9
  x : Outport  Port=10
  y : Outport  Port=11
  H : Outport  Port=12
  mach : Outport  Port=13
  gamma : Outport  Port=14
  chi : Outport  Port=15
  Vy : Outport  Port=16
  nyb : Outport  Port=17
  nzb : Outport  Port=18
  Acc : Outport  Port=19
  Ve : Outport  Port=20
  To : Outport  Port=21
  Po : Outport  Port=22
  nb : Outport  Port=23
  wires:
  Bus Selector/9 -> Radians to Degrees/1  "<gamma>"
  Bus Selector/8 -> Radians to Degrees1/1  "<pqr>"
  Bus Selector/7 -> Radians to Degrees2/1  "<beta>"
  Bus Selector/5 -> [V]  "<Va>"
  Bus Selector/2 -> [nb]  "<nb>"
  Bus Selector/1 -> Radians to Degrees4/1  "<Euler>"
  Bus Selector/6 -> Radians to Degrees3/1  "<alpha>"
  Bus Selector/4 -> [Xe]  "<Xe>"
  Model o/p bus/1 -> Bus Selector/1
  Bus Selector/3 -> [Mach]  "<mach>"
  Bus Selector/11 -> [Ve]  "<Ve>"
  6/1 -> q/1
  9/1 -> p/1
  [pqr] -> 6/1, 9/1, 10/1
  10/1 -> r/1
  [Euler] -> 4/1, 1/1, 2/1
  4/1 -> psi/1
  2/1 -> phi/1
  1/1 -> theta/1
  [alpha] -> alpha/1
  [beta] -> beta/1
  14/1 -> y/1
  Gain/1 -> H/1
  11/1 -> Gain/1
  [Xe] -> 11/1, 14/1, 7/1
  [Mach] -> mach/1
  [gamma] -> gamma/1
  Gain1/1 -> Vy/1
  5/1 -> Gain1/1
  [Ve] -> 5/1
  7/1 -> x/1
  [V] -> Va/1
  Radians to Degrees/1 -> [gamma]
  Radians to Degrees1/1 -> [pqr]
  Radians to Degrees2/1 -> [beta]
  Radians to Degrees3/1 -> [alpha]
  Radians to Degrees4/1 -> [Euler]
  [nb] -> nb/1, 8/1, 3/1
  8/1 -> nyb/1
  3/1 -> nzb/1
  Bus Selector/10 -> Radians to Degrees5/1  "<chi>"
  Radians to Degrees5/1 -> [chi]
  [chi] -> chi/1
  Bus Selector/12 -> [Acc]  "<Accels>"
  [Acc] -> Acc/1
  [Ve] -> Ve/1
  Bus Selector/13 -> [To]  "<To>"
  Bus Selector/14 -> [Po]  "<Po>"
  [Po] -> Po/1
  [To] -> To/1

== system SIMQGC/Controller/RAH ==
  Phic : Inport
  phi : Inport  Port=2
  p : Inport  Port=3
  r : Inport  Port=4
  ayb : Inport  Port=5
  Gain : Gain  Gain=Kphi
  Gain1 : Gain  Gain=Kp
  Gain2 : Gain  Gain=Kr
  Gain3 : Gain  Gain=Kay
  Gain4 : Gain  Gain=Kff_phi
  Gain5 : Gain  Gain=Kpi
  Integrator : Integrator
  Sum : Sum  Inputs=|+-
  Sum1 : Sum  Inputs=|-+
  Sum2 : Sum  Inputs=-+++
  Sum3 : Sum  Inputs=|++
  dd : Outport
  wires:
  Phic/1 -> Gain4/1, Sum/1
  phi/1 -> Sum/2
  Sum/1 -> Gain/1
  p/1 -> Sum1/2
  Gain/1 -> Sum1/1
  Sum1/1 -> Gain5/1, Gain1/1
  Gain2/1 -> Sum2/3
  Gain3/1 -> Sum2/4
  Sum2/1 -> dd/1
  Gain4/1 -> Sum2/1
  ayb/1 -> Gain3/1
  Gain1/1 -> Sum3/1
  Sum3/1 -> Sum2/2
  Integrator/1 -> Sum3/2
  Gain5/1 -> Integrator/1
  r/1 -> Gain2/1

== system SIMQGC/Controller/Subsystem ==
  In1 : Inport
  Gain7 : Gain  Gain=0.1
  Gain8 : Gain
  Integrator : Integrator  LimitOutput=on  UpperSaturationLimit=10  LowerSaturationLimit=-10
  Memory : Memory
  Saturation : Saturate  UpperLimit=10  LowerLimit=-10
  Sum1 : Sum  Inputs=++|  SaturateOnIntegerOverflow=on
  Out1 : Outport
  wires:
  In1/1 -> Gain7/1, Gain8/1
  Saturation/1 -> Memory/1  "thetac(deg)"
  Gain7/1 -> Integrator/1
  Gain8/1 -> Sum1/1
  Sum1/1 -> Saturation/1
  Integrator/1 -> Sum1/2
  Memory/1 -> Out1/1

== system SIMQGC/Controller/height_hold ==
  note: height hold
  Hc : Inport
  H : Inport  Port=2
  Add : Sum  Inputs=|+-
  Gain1 : Gain  Gain=0.1
  Gain4 : Gain
  Integrator : Integrator  LimitOutput=on  UpperSaturationLimit=10  LowerSaturationLimit=-10
  Saturation : Saturate  UpperLimit=10  LowerLimit=-10
  Sum1 : Sum  Inputs=++|  SaturateOnIntegerOverflow=on
  thetac : Outport
  wires:
  Saturation/1 -> thetac/1  "thetac(deg)"
  Sum1/1 -> Saturation/1
  H/1 -> Add/2
  Gain1/1 -> Integrator/1
  Gain4/1 -> Sum1/1
  Hc/1 -> Add/1
  Integrator/1 -> Sum1/2
  Add/1 -> Gain1/1, Gain4/1

== system SIMQGC/Controller/theta_hold ==
  note: theta hold
  thetac : Inport
  theta : Inport  Port=2
  q : Inport  Port=3
  Add : Sum  Inputs=|+-
  Gain : Gain  Gain=0.1
  Gain1 : Gain
  Gain4 : Gain
  Gain5 : Gain  Gain=0
  Integrator : Integrator
  Memory1 : Memory
  Sum1 : Sum  Inputs=-+  SaturateOnIntegerOverflow=on
  Sum2 : Sum  Inputs=|++  SaturateOnIntegerOverflow=on
  de : Outport
  wires:
  thetac/1 -> Add/1
  q/1 -> Gain5/1
  theta/1 -> Add/2
  Gain4/1 -> Sum1/1
  Gain5/1 -> Sum1/2
  Sum1/1 -> Gain1/1, Gain/1
  Gain/1 -> Sum2/1
  Integrator/1 -> Sum2/2
  Gain1/1 -> Integrator/1
  Sum2/1 -> Memory1/1
  Add/1 -> Gain4/1
  Memory1/1 -> de/1

== system SIMQGC/Controller/v_hold1 ==
  note: height hold
  Va : Inport
  Vc : Inport  Port=2
  Add : Sum  Inputs=|+-
  Gain1 : Gain  Gain=0.1
  Gain4 : Gain
  Integrator : Integrator  LimitOutput=on  UpperSaturationLimit=10  LowerSaturationLimit=-10
  Memory1 : Memory
  Saturation : Saturate  UpperLimit=10  LowerLimit=-10
  Sum1 : Sum  Inputs=++|  SaturateOnIntegerOverflow=on
  tg : Outport
  wires:
  Saturation/1 -> Memory1/1  "thetac(deg)"
  Sum1/1 -> Saturation/1
  Vc/1 -> Add/2
  Gain1/1 -> Integrator/1
  Gain4/1 -> Sum1/1
  Va/1 -> Add/1
  Integrator/1 -> Sum1/2
  Add/1 -> Gain1/1, Gain4/1
  Memory1/1 -> tg/1

== system SIMQGC/UDPReadFromQGC/Subsystem ==
  note: Normed to -1..+1 where 0 is neutral position. Throttle for single rotation direction motors is 0..1,
      | negative range for reverse direction. Standard mapping for attitude controls (group 0):
      |  (index 0-7): roll, pitch, yaw, throttle, flaps, spoilers, airbrakes, landing gear. Load a pass-through mixer to repurpose them as generic outputs.
  msg : Inport
  length : Inport  Port=2
  Demux : Demux  Outputs=3
  Demux1 : Demux  Outputs=2
  MATLAB Function : MATLAB Function  TreatAsAtomicUnit=on
  Scope : Scope
  Scope1 : Scope  NumInputPorts=2
  Switch Case : SwitchCase  CaseConditions={8,25}
  Terminator : Terminator
  data_transfer : MATLAB Function  TreatAsAtomicUnit=on
  joystick : Subsystem  TreatAsAtomicUnit=on
  throttle : Subsystem  TreatAsAtomicUnit=on
  thro1_part : Outport
  thro2_part : Outport  Port=2
  elev_yoke : Outport  Port=3
  ailrn_yoke : Outport  Port=4
  ruddr_yoke : Outport  Port=5
  wires:
  Switch Case/1 -> joystick/Action
  data_transfer/1(index) -> Switch Case/1, Scope/1
  data_transfer/2(control) -> throttle/1(data), joystick/1(data)
  Demux1/1 -> Scope1/1, thro1_part/1
  joystick/1(joystick) -> Demux/1
  Switch Case/2 -> throttle/Action
  Demux/2 -> ailrn_yoke/1
  Switch Case/3 -> Terminator/1
  Demux/3 -> ruddr_yoke/1
  Demux/1 -> elev_yoke/1
  MATLAB Function/1(data) -> data_transfer/1(data)
  msg/1 -> MATLAB Function/1(a)
  length/1 -> MATLAB Function/2(length)
  throttle/1(throttle) -> Demux1/1
  Demux1/2 -> Scope1/2, thro2_part/1

== system SIMQGC/UDPSendToQGC/UDP_send 16 ==
  Q_rad_s : Inport
  P_rad_s : Inport  Port=2
  R_rad_s : Inport  Port=3
  Byte Pack : MATLAB Function  TreatAsAtomicUnit=on
  Gain : Gain  Gain=pi/180
  Mux : Mux  Inputs=8
  Null3 : Constant  Value=0
  UDP send 16 : dspnetwork/UDP Send  remoteURL='127.0.0.1'  remotePort=49005  localURL='0.0.0.0'  localPortSource=Automatically determine  localPort=-1  sampletime=-1  blockPlatform=HOST  separateLengthPort=0
  Vind_keas : Constant  Value=0
  Vind_kias : Constant  Value=0
  Vtrue_ktas : Constant  Value=0
  Vtrue_ktgs : Constant  Value=0
  head : Constant  Value=[68,65,84,65,64]  OutDataTypeStr=fixdt('uint8', 'DataTypeOverride', 'Off')
  index : Constant  Value=16  OutDataTypeStr=fixdt('uint8', 'DataTypeOverride', 'Off')
  wires:
  Mux/1 -> Gain/1
  Vtrue_ktgs/1 -> Mux/4
  Byte Pack/1(OUT) -> UDP send 16/1
  head/1 -> Byte Pack/1(head)  "head"
  index/1 -> Byte Pack/2(index)  "index"
  Vtrue_ktas/1 -> Mux/5
  Null3/1 -> Mux/8
  Vind_keas/1 -> Mux/7
  Vind_kias/1 -> Mux/6
  P_rad_s/1 -> Mux/2
  Q_rad_s/1 -> Mux/1
  R_rad_s/1 -> Mux/3
  Gain/1 -> Byte Pack/3(data)

== system SIMQGC/UDPSendToQGC/UDP_send 17 ==
  pitch_deg : Inport
  roll_deg : Inport  Port=2
  hding_true : Inport  Port=3
  hding_mag : Inport  Port=4
  Byte Pack : MATLAB Function  TreatAsAtomicUnit=on
  Mux : Mux  Inputs=8
  Null3 : Constant  Value=0
  UDP send 17 : dspnetwork/UDP Send  remoteURL='127.0.0.1'  remotePort=49005  localURL='0.0.0.0'  localPortSource=Automatically determine  localPort=-1  sampletime=-1  blockPlatform=HOST  separateLengthPort=0
  Vind_keas : Constant  Value=0
  Vind_kias : Constant  Value=0
  Vtrue_ktas : Constant  Value=0
  head : Constant  Value=[68,65,84,65,64]  OutDataTypeStr=fixdt('uint8', 'DataTypeOverride', 'Off')
  index : Constant  Value=17  OutDataTypeStr=fixdt('uint8', 'DataTypeOverride', 'Off')
  wires:
  Byte Pack/1(OUT) -> UDP send 17/1
  head/1 -> Byte Pack/1(head)  "head"
  index/1 -> Byte Pack/2(index)  "index"
  Vtrue_ktas/1 -> Mux/5
  Null3/1 -> Mux/8
  Vind_keas/1 -> Mux/7
  Vind_kias/1 -> Mux/6
  roll_deg/1 -> Mux/2
  pitch_deg/1 -> Mux/1
  hding_true/1 -> Mux/3
  Mux/1 -> Byte Pack/3(data)
  hding_mag/1 -> Mux/4

== system SIMQGC/UDPSendToQGC/UDP_send 20 ==
  lat_deg : Inport
  lon_deg : Inport  Port=2
  alt_ftmsl : Inport  Port=3
  alt_ftagl : Inport  Port=4
  Byte Pack : MATLAB Function  TreatAsAtomicUnit=on
  Gain : Gain  Gain=3.280839895013
  Gain1 : Gain  Gain=3.280839895013
  Mux : Mux  Inputs=8
  Null3 : Constant  Value=0
  UDP send 20 : dspnetwork/UDP Send  remoteURL='127.0.0.1'  remotePort=49005  localURL='0.0.0.0'  localPortSource=Automatically determine  localPort=-1  sampletime=-1  blockPlatform=HOST  separateLengthPort=0
  Vind_keas : Constant  Value=0
  Vind_kias : Constant  Value=0
  Vtrue_ktas : Constant  Value=0
  head : Constant  Value=[68,65,84,65,64]  OutDataTypeStr=fixdt('uint8', 'DataTypeOverride', 'Off')
  index : Constant  Value=20  OutDataTypeStr=fixdt('uint8', 'DataTypeOverride', 'Off')
  wires:
  Byte Pack/1(OUT) -> UDP send 20/1
  head/1 -> Byte Pack/1(head)  "head"
  index/1 -> Byte Pack/2(index)  "index"
  Vtrue_ktas/1 -> Mux/5
  Null3/1 -> Mux/8
  Vind_keas/1 -> Mux/7
  Vind_kias/1 -> Mux/6
  lon_deg/1 -> Mux/2
  lat_deg/1 -> Mux/1
  alt_ftmsl/1 -> Gain/1
  Mux/1 -> Byte Pack/3(data)
  alt_ftagl/1 -> Gain1/1
  Gain/1 -> Mux/3
  Gain1/1 -> Mux/4

== system SIMQGC/UDPSendToQGC/UDP_send 21 ==
  vX_m_s : Inport
  vY_m_s : Inport  Port=2
  vZ_m_s : Inport  Port=3
  Byte Pack : MATLAB Function  TreatAsAtomicUnit=on
  Gain : Gain  Gain=-1
  Gain1 : Gain  Gain=-1
  Mux : Mux  Inputs=8
  Null3 : Constant  Value=0
  UDP send 21 : dspnetwork/UDP Send  remoteURL='127.0.0.1'  remotePort=49005  localURL='0.0.0.0'  localPortSource=Automatically determine  localPort=-1  sampletime=-1  blockPlatform=HOST  separateLengthPort=0
  Vind_keas : Constant  Value=0
  Vind_kias : Constant  Value=0
  Vtrue_ktas : Constant  Value=0
  Vtrue_ktgs : Constant  Value=0
  head : Constant  Value=[68,65,84,65,64]  OutDataTypeStr=fixdt('uint8', 'DataTypeOverride', 'Off')
  index : Constant  Value=21  OutDataTypeStr=fixdt('uint8', 'DataTypeOverride', 'Off')
  wires:
  Mux/1 -> Byte Pack/3(data)
  Byte Pack/1(OUT) -> UDP send 21/1
  head/1 -> Byte Pack/1(head)  "head"
  index/1 -> Byte Pack/2(index)  "index"
  Null3/1 -> Mux/8
  vX_m_s/1 -> Gain1/1
  vZ_m_s/1 -> Gain/1
  Vind_kias/1 -> Mux/1
  Vtrue_ktas/1 -> Mux/2
  Vtrue_ktgs/1 -> Mux/3
  Gain/1 -> Mux/6
  Vind_keas/1 -> Mux/7
  vY_m_s/1 -> Mux/5
  Gain1/1 -> Mux/4

== system SIMQGC/UDPSendToQGC/UDP_send 3  ==
  Vind_mph : Inport
  Vtrue_mphas : Inport  Port=2
  Vtrue_mphgs : Inport  Port=3
  Byte Pack : MATLAB Function  TreatAsAtomicUnit=on
  Gain : Gain  Gain=1/0.5144
  Mux : Mux  Inputs=8
  Null3 : Constant  Value=999
  UDP send 3 : dspnetwork/UDP Send  remoteURL='127.0.0.1'  remotePort=49005  localURL='0.0.0.0'  localPortSource=Automatically determine  localPort=-1  sampletime=-1  blockPlatform=HOST  separateLengthPort=0
  Vind_keas : Constant  Commented=on  Value=0
  Vind_kias : Constant  Commented=on  Value=0
  Vtrue_ktas : Constant  Commented=on  Value=0
  Vtrue_ktgs : Constant  Commented=on  Value=0
  head : Constant  Value=[68,65,84,65,64]  OutDataTypeStr=fixdt('uint8', 'DataTypeOverride', 'Off')
  index : Constant  Value=3  OutDataTypeStr=fixdt('uint8', 'DataTypeOverride', 'Off')
  wires:
  Vtrue_mphas/1 -> Mux/7
  Null3/1 -> Mux/5
  Mux/1 -> Gain/1
  Vtrue_mphgs/1 -> Mux/8
  Vind_mph/1 -> Mux/1, Mux/2, Mux/3, Mux/4, Mux/6
  Byte Pack/1(OUT) -> UDP send 3/1
  head/1 -> Byte Pack/1(head)  "head"
  index/1 -> Byte Pack/2(index)  "index"
  Gain/1 -> Byte Pack/3(data)

== system SIMQGC/UDPSendToQGC/UDP_send 4 ==
  Gload_nomal : Inport
  Gload_axial : Inport  Port=2
  Gload_side : Inport  Port=3
  Byte Pack : MATLAB Function  TreatAsAtomicUnit=on
  Mux : Mux  Inputs=8
  Null3 : Constant  Value=0
  UDP send 4 : dspnetwork/UDP Send  remoteURL='127.0.0.1'  remotePort=49005  localURL='0.0.0.0'  localPortSource=Automatically determine  localPort=-1  sampletime=-1  blockPlatform=HOST  separateLengthPort=0
  Vind_keas : Constant  Value=0
  Vind_kias : Constant  Value=0
  Vtrue_ktas : Constant  Value=0
  Vtrue_ktgs : Constant  Value=0
  head : Constant  Value=[68,65,84,65,64]  OutDataTypeStr=fixdt('uint8', 'DataTypeOverride', 'Off')
  index : Constant  Value=4  OutDataTypeStr=fixdt('uint8', 'DataTypeOverride', 'Off')
  wires:
  Vind_kias/1 -> Mux/1
  Vtrue_ktgs/1 -> Mux/4
  Vind_keas/1 -> Mux/2
  Gload_axial/1 -> Mux/6
  Byte Pack/1(OUT) -> UDP send 4/1
  head/1 -> Byte Pack/1(head)  "head"
  index/1 -> Byte Pack/2(index)  "index"
  Vtrue_ktas/1 -> Mux/3
  Null3/1 -> Mux/8
  Mux/1 -> Byte Pack/3(data)
  Gload_side/1 -> Mux/7
  Gload_nomal/1 -> Mux/5

== system SIMQGC/UDPSendToQGC/UDP_send 6 ==
  AMprs_inHG : Inport
  AMtmp_degC : Inport  Port=2
  Add : Sum  Inputs=+-
  Byte Pack : MATLAB Function  TreatAsAtomicUnit=on
  Constant : Constant  Value=273.15
  Mux : Mux  Inputs=8
  Null3 : Constant  Value=0
  UDP send 6 : dspnetwork/UDP Send  remoteURL='127.0.0.1'  remotePort=49005  localURL='0.0.0.0'  localPortSource=Automatically determine  localPort=-1  sampletime=-1  blockPlatform=HOST  separateLengthPort=0
  Vind_keas : Constant  Value=0
  Vind_kias : Constant  Value=0
  Vtrue_ktas : Constant  Value=0
  Vtrue_ktgs : Constant  Value=0
  Vtrue_ktgs1 : Constant  Value=0
  head : Constant  Value=[68,65,84,65,64]  OutDataTypeStr=fixdt('uint8', 'DataTypeOverride', 'Off')
  index : Constant  Value=6  OutDataTypeStr=fixdt('uint8', 'DataTypeOverride', 'Off')
  pa->in Hg : Gain  Gain=1/3386.3881579
  wires:
  Mux/1 -> Byte Pack/3(data)
  Vtrue_ktgs/1 -> Mux/4
  Byte Pack/1(OUT) -> UDP send 6/1
  head/1 -> Byte Pack/1(head)  "head"
  index/1 -> Byte Pack/2(index)  "index"
  Vtrue_ktas/1 -> Mux/3
  Null3/1 -> Mux/8
  Vind_keas/1 -> Mux/7
  Vind_kias/1 -> Mux/6
  AMtmp_degC/1 -> Add/1
  AMprs_inHG/1 -> pa->in Hg/1
  pa->in Hg/1 -> Mux/1
  Vtrue_ktgs1/1 -> Mux/5
  Constant/1 -> Add/2
  Add/1 -> Mux/2

== system SIMQGC/toUDP/Subsystem ==
  In1 : Inport
  Demux : Demux  Outputs=3
  Mux1 : Mux  Inputs=3
  Transfer Fcn : TransferFcn  Denominator=[1 1]
  Transfer Fcn2 : TransferFcn  Denominator=[1 1]
  Transfer Fcn3 : TransferFcn  Denominator=[1 1]
  Out1 : Outport
  wires:
  Transfer Fcn3/1 -> Mux1/3
  Demux/2 -> Transfer Fcn2/1
  Demux/1 -> Transfer Fcn/1
  In1/1 -> Demux/1
  Transfer Fcn2/1 -> Mux1/2
  Mux1/1 -> Out1/1
  Transfer Fcn/1 -> Mux1/1
  Demux/3 -> Transfer Fcn3/1

== system SIMQGC/toUDP/Subsystem1 ==
  In1 : Inport
  Demux : Demux  Outputs=3
  Mux1 : Mux  Inputs=3
  Transfer Fcn : TransferFcn  Denominator=[1 1]
  Transfer Fcn2 : TransferFcn  Denominator=[1 1]
  Transfer Fcn3 : TransferFcn  Denominator=[1 1]
  Out1 : Outport
  wires:
  Demux/3 -> Transfer Fcn3/1
  Transfer Fcn/1 -> Mux1/1
  Mux1/1 -> Out1/1
  Transfer Fcn2/1 -> Mux1/2
  In1/1 -> Demux/1
  Demux/1 -> Transfer Fcn/1
  Demux/2 -> Transfer Fcn2/1
  Transfer Fcn3/1 -> Mux1/3

== system SIMQGC/toUDP/Subsystem2 ==
  vin : Inport
  Sum : Sum  Inputs=|+-
  Wrap To Zero : simulink/Discontinuities/Wrap To Zero  Threshold=t
      settings: SourceProductName=Simulink  SourceProductBaseCode=SL
  vout : Outport
  wires:
  Wrap To Zero/1 -> Sum/2
  Sum/1 -> vout/1
  vin/1 -> Wrap To Zero/1, Sum/1

== system SIMQGC/toUDP/Subsystem3 ==
  vin : Inport
  Sum : Sum  Inputs=|+-
  Wrap To Zero : simulink/Discontinuities/Wrap To Zero  Threshold=t
      settings: SourceProductName=Simulink  SourceProductBaseCode=SL
  vout : Outport
  wires:
  vin/1 -> Sum/1, Wrap To Zero/1
  Sum/1 -> vout/1
  Wrap To Zero/1 -> Sum/2

== system SIMQGC/toUDP/Subsystem4 ==
  vin : Inport
  Sum : Sum  Inputs=|+-
  Wrap To Zero : simulink/Discontinuities/Wrap To Zero  Threshold=t
      settings: SourceProductName=Simulink  SourceProductBaseCode=SL
  vout : Outport
  wires:
  Wrap To Zero/1 -> Sum/2
  Sum/1 -> vout/1
  vin/1 -> Wrap To Zero/1, Sum/1

== system SIMQGC/toUDP/Subsystem5 ==
  vin : Inport
  Sum : Sum  Inputs=|+-
  Wrap To Zero : simulink/Discontinuities/Wrap To Zero  Threshold=t
      settings: SourceProductName=Simulink  SourceProductBaseCode=SL
  vout : Outport
  wires:
  vin/1 -> Sum/1, Wrap To Zero/1
  Sum/1 -> vout/1
  Wrap To Zero/1 -> Sum/2
